simulink model "RobotArmVersion4Assem"  (R2025b)
(part 2 of 11)

  Cylindrical22/LConn1 -- Robot_Arm_2_Version_4_1_RIGID/RConn4
  Cylindrical22/RConn1 -- Motor_Enclosure_Assem_5/LConn1
  Planar18/LConn1 -- Robot_Arm_2_Version_4_1_RIGID/RConn2
  Planar18/RConn1 -- SS_joint_shaft_3_Quarter_Diameter_1_RIGID/LConn2
  x18_Tooth_Timing_Belt_Pulley_1326N51_1_RIGID/LConn3 -- x48_Tooth_Timing_Belt_Pulley_1326N63_1_RIGID/LConn2
  Revolute13/LConn1 -- Robot_Arm_1_Curved_Version_4_3_RIGID/RConn17
  Cylindrical3/RConn1 -- x6436K71_Clamping_Two_Piece_Shaft_Collar_3_RIGID/LConn1
  Revolute13/RConn1 -- x18_Tooth_Timing_Belt_Pulley_1326N51_1_RIGID/LConn1
  Tension_belt_mockup_with_tensioner_2_RIGID/LConn2 -- x18_Tooth_Timing_Belt_Pulley_1326N51_1_RIGID/LConn2
  Arm_Hitch_Track_Rod_Prototype_1_RIGID/LConn1 -- Transform1/RConn1
  Cylindrical23/LConn1 -- x98957A184_Grade_B7_Medium_Strength_Steel_Threaded_Rod_1_RIGID/RConn2
  Cylindrical23/RConn1 -- x2796T14_Ultra_Low_Friction_Dry_Running_Thrust_Bearing_1_RIGID/LConn1
  Revolute14/LConn1 -- SS_joint_shaft_3_Quarter_Diameter_1_RIGID/RConn1
  Revolute14/RConn1 -- x6436K72_Clamping_Two_Piece_Shaft_Collar_1_RIGID/LConn2
  Cylindrical24/LConn1 -- SS_joint_shaft_3_Quarter_Diameter_1_RIGID/RConn2
  Cylindrical24/RConn1 -- x6436K72_Clamping_Two_Piece_Shaft_Collar_2_RIGID/LConn1
  Arm_Hitch_Track_Rod_Prototype_1_RIGID/RConn2 -- Planar19/LConn1
  Planar2/LConn1 -- x6436K71_Clamping_Two_Piece_Shaft_Collar_3_RIGID/RConn1
  Arm_Hitch_Track_Rod_Prototype_2_RIGID/LConn2 -- Planar19/RConn1
  Arm_Hitch_Track_Rod_Prototype_1_RIGID/RConn4 -- Planar20/LConn1
  Arm_Hitch_Track_Rod_Prototype_4_RIGID/LConn2 -- Planar20/RConn1
  Arm_Hitch_Track_Rod_Prototype_1_RIGID/RConn3 -- Revolute15/LConn1
  Arm_Base_Mount_Clamp_Motor_Mount_Assem_4_RIGID/LConn2 -- Revolute15/RConn1
  Arm_Hitch_Track_Rod_Prototype_2_RIGID/RConn1 -- Planar21/LConn1
  Arm_Hitch_Track_Rod_Prototype_3_RIGID/LConn2 -- Planar21/RConn1
  Arm_Hitch_Track_Rod_Prototype_2_RIGID/RConn2 -- Cylindrical25/LConn1
  Arm_Base_Mount_Clamp_Motor_Mount_Assem_4_RIGID/LConn1 -- Cylindrical25/RConn1
  Arm_Base_Mount_Clamp_Motor_Mount_Assem_4_RIGID/RConn2 -- Cylindrical26/LConn1
  Planar2/RConn1 -- Robot_Arm_1_Curved_Version_4_3_RIGID/LConn2
  Arm_Hitch_Track_Rod_Prototype_3_RIGID/LConn1 -- Cylindrical26/RConn1
  Arm_Base_Mount_Clamp_Motor_Mount_Assem_4_RIGID/RConn4 -- Cylindrical27/LConn1
  Arm_Hitch_Track_Rod_Prototype_4_RIGID/LConn1 -- Cylindrical27/RConn1
  Arm_Base_Mount_Clamp_Motor_Mount_Assem_4_RIGID/RConn1 -- Cylindrical28/LConn1
  Cylindrical28/RConn1 -- Motor_Enclosure_Assem_6/LConn1
  Planar22/LConn1 -- x6443K42_Single_U_Joint_1_RIGID/RConn1
  Motor_Enclosure_Assem_6/LConn3 -- Planar22/RConn1
  Revolute16/LConn1 -- x98957A184_Grade_B7_Medium_Strength_Steel_Threaded_Rod_1_RIGID/RConn1
  Revolute16/RConn1 -- x6443K42_Single_U_Joint_1_RIGID/LConn1
  Chuck_Mount_Assem_1/RConn1 -- Cylindrical29/LConn1
  Cylindrical4/LConn1 -- SS_joint_shaft_3_RIGID/RConn1
  Cylindrical29/RConn1 -- Robot_Arm_2_Version_4_1_RIGID/LConn1
  Arm_Hitch_Version_4_2_RIGID/RConn19 -- Cylindrical30/LConn1
  Cylindrical30/RConn1 -- Motor_Enclosure_Assem_4/LConn3
  Revolute17/LConn1 -- x48_Tooth_Timing_Belt_Pulley_1326N63_1_RIGID/RConn1
  Revolute17/RConn1 -- Tension_belt_mockup_with_tensioner_2_RIGID/LConn1
  Arm_Hitch_Version_4_2_RIGID/RConn22 -- Planar23/LConn1
  Planar23/RConn1 -- x6436K71_Clamping_Two_Piece_Shaft_Collar_8_RIGID/LConn2
  Arm_Hitch_Version_4_2_RIGID/RConn23 -- Planar24/LConn1
  Planar24/RConn1 -- SS_joint_shaft_1_RIGID/LConn2
  Arm_Hitch_Version_4_2_RIGID/RConn7 -- Planar25/LConn1
  Cylindrical4/RConn1 -- x6436K71_Clamping_Two_Piece_Shaft_Collar_4_RIGID/LConn2
  Planar25/RConn1 -- SS_joint_shaft_2_RIGID/LConn1
  Arm_Hitch_Version_4_2_RIGID/RConn5 -- Planar26/LConn1
  Planar26/RConn1 -- SS_joint_shaft_3_RIGID/LConn1
  Arm_Hitch_Version_4_2_RIGID/RConn6 -- Planar27/LConn1
  Planar27/RConn1 -- SS_joint_shaft_4_RIGID/LConn2
  Arm_Hitch_Version_4_2_RIGID/RConn4 -- Revolute18/LConn1
  Revolute18/RConn1 -- SS_joint_shaft_5_RIGID/LConn1
  Arm_Hitch_Version_4_2_RIGID/RConn3 -- Planar28/LConn1
  Planar28/RConn1 -- x6436K71_Clamping_Two_Piece_Shaft_Collar_11_RIGID/LConn2
  Arm_Hitch_Version_4_2_RIGID/RConn1 -- Revolute19/LConn1
  Planar3/LConn1 -- x1258N17_11_8_OD_PEEK_Plastic_Ball_Bearing_1_RIGID/RConn1
  Revolute19/RConn1 -- Robot_Arm_1_Curved_Version_4_3_RIGID/LConn1
  Arm_Hitch_Version_4_2_RIGID/RConn2 -- Planar29/LConn1
  Motor_Enclosure_Assem_4/LConn1 -- Planar29/RConn1
  Arm_Hitch_Version_4_2_RIGID/RConn21 -- Revolute20/LConn1
  Revolute20/RConn1 -- x1258N23_15_8_OD_PEEK_Plastic_Ball_Bearing_4_RIGID/LConn1
  Revolute21/LConn1 -- x9533T3_Self_Aligning_Linear_Sleeve_Bearing_1_RIGID/RConn1
  Arm_Hitch_Version_4_2_RIGID/LConn2 -- Revolute21/RConn1
  Arm_Hitch_Version_4_2_RIGID/RConn20 -- Revolute22/LConn1
  Revolute22/RConn1 -- x9533T3_Self_Aligning_Linear_Sleeve_Bearing_2_RIGID/LConn1
  Arm_Hitch_Version_4_2_RIGID/RConn18 -- Revolute23/LConn1
  Planar3/RConn1 -- x6436K71_Clamping_Two_Piece_Shaft_Collar_4_RIGID/LConn1
  Revolute23/RConn1 -- x9533T3_Self_Aligning_Linear_Sleeve_Bearing_3_RIGID/LConn1
  Arm_Hitch_Version_4_2_RIGID/RConn17 -- Revolute24/LConn1
  Revolute24/RConn1 -- x9533T3_Self_Aligning_Linear_Sleeve_Bearing_4_RIGID/LConn1
  Arm_Hitch_Version_4_2_RIGID/RConn16 -- Revolute25/LConn1
  Revolute25/RConn1 -- x9533T3_Self_Aligning_Linear_Sleeve_Bearing_5_RIGID/LConn1
  Arm_Hitch_Version_4_2_RIGID/RConn14 -- Revolute26/LConn1
  Revolute26/RConn1 -- x9533T3_Self_Aligning_Linear_Sleeve_Bearing_6_RIGID/LConn1
  Arm_Hitch_Version_4_2_RIGID/RConn12 -- Revolute27/LConn1
  Revolute27/RConn1 -- x9533T3_Self_Aligning_Linear_Sleeve_Bearing_7_RIGID/LConn1
  Arm_Hitch_Version_4_2_RIGID/RConn11 -- Revolute28/LConn1
  Cylindrical5/LConn1 -- SS_joint_shaft_1_RIGID/RConn2
  Revolute28/RConn1 -- x9533T3_Self_Aligning_Linear_Sleeve_Bearing_8_RIGID/LConn1
  Arm_Hitch_Version_4_2_RIGID/RConn10 -- Revolute29/LConn1
  PEEK_Thread_Insert_1_RIGID/LConn1 -- Revolute29/RConn1
  Arm_Hitch_Version_4_2_RIGID/RConn9 -- Rectangular/LConn1
  Rectangular/RConn1 -- Transform2/RConn1
  Arm_Hitch_Version_4_2_RIGID/RConn8 -- Cylindrical31/LConn1
  Cylindrical31/RConn1 -- Motor_Enclosure_Assem_4/LConn2
  Arm_Hitch_Track_Rod_Prototype_1_RIGID/RConn1 -- Cylindrical32/LConn1
  Arm_Hitch_Version_4_2_RIGID/LConn1 -- Cylindrical32/RConn1
  Arm_Hitch_Version_4_2_RIGID/RConn15 -- Cylindrical33/LConn1
  Cylindrical/RConn1 -- Motor_Enclosure_Assem_5/LConn3
  Cylindrical5/RConn1 -- x6436K71_Clamping_Two_Piece_Shaft_Collar_5_RIGID/LConn1
  Arm_Hitch_Track_Rod_Prototype_2_RIGID/LConn1 -- Cylindrical33/RConn1
  Arm_Hitch_Version_4_2_RIGID/RConn13 -- Revolute30/LConn1
  Arm_Linkage_1_3_RIGID/LConn1 -- Revolute30/RConn1
  Arm_Linkage_1_3_RIGID/RConn2 -- Cylindrical34/LConn1
  Arm_Linkage_2_2_RIGID/LConn2 -- Cylindrical34/RConn1
  Arm_Linkage_1_3_RIGID/RConn1 -- Cylindrical35/LConn1
  Arm_Linkage_2_3_RIGID/LConn2 -- Cylindrical35/RConn1
  Revolute31/LConn1 -- Robot_Arm_1_Curved_Version_4_3_RIGID/RConn12
  Arm_Linkage_2_2_RIGID/LConn1 -- Revolute31/RConn1
  Arm_Linkage_2_2_RIGID/RConn2 -- Revolute32/LConn1
  Planar4/LConn1 -- x6436K71_Clamping_Two_Piece_Shaft_Collar_5_RIGID/RConn1
  Revolute32/RConn1 -- x1258N17_11_8_OD_PEEK_Plastic_Ball_Bearing_3_RIGID/LConn1
  Arm_Linkage_2_2_RIGID/RConn1 -- Revolute33/LConn1
  Revolute33/RConn1 -- x1258N17_11_8_OD_PEEK_Plastic_Ball_Bearing_6_RIGID/LConn1
  Revolute34/LConn1 -- Robot_Arm_1_Curved_Version_4_3_RIGID/RConn11
  Arm_Linkage_2_3_RIGID/LConn1 -- Revolute34/RConn1
  Arm_Linkage_2_3_RIGID/RConn1 -- Revolute35/LConn1
  Revolute35/RConn1 -- x1258N17_11_8_OD_PEEK_Plastic_Ball_Bearing_1_RIGID/LConn1
  Arm_Linkage_2_3_RIGID/RConn2 -- Revolute36/LConn1
  Revolute36/RConn1 -- x1258N17_11_8_OD_PEEK_Plastic_Ball_Bearing_5_RIGID/LConn1
  Planar4/RConn1 -- x1258N17_11_8_OD_PEEK_Plastic_Ball_Bearing_6_RIGID/LConn2
  Cylindrical6/LConn1 -- SS_joint_shaft_1_RIGID/RConn1
  Cylindrical6/RConn1 -- x6436K71_Clamping_Two_Piece_Shaft_Collar_6_RIGID/LConn1
  Planar5/LConn1 -- x6436K71_Clamping_Two_Piece_Shaft_Collar_6_RIGID/RConn1
  Planar5/RConn1 -- x1258N17_11_8_OD_PEEK_Plastic_Ball_Bearing_5_RIGID/LConn2
  Cylindrical7/LConn1 -- SS_joint_shaft_5_RIGID/RConn2
  Cylindrical7/RConn1 -- x6436K71_Clamping_Two_Piece_Shaft_Collar_8_RIGID/LConn1
  Cylindrical8/LConn1 -- SS_joint_shaft_4_RIGID/RConn2
  Cylindrical1/LConn1 -- x6436K71_Clamping_Two_Piece_Shaft_Collar_1_RIGID/RConn1
  Cylindrical8/RConn1 -- x6436K71_Clamping_Two_Piece_Shaft_Collar_9_RIGID/LConn1
  Planar6/LConn1 -- Robot_Arm_1_Curved_Version_4_3_RIGID/RConn16
  Planar6/RConn1 -- x6436K71_Clamping_Two_Piece_Shaft_Collar_9_RIGID/LConn2
  Cylindrical9/LConn1 -- x1258N17_11_8_OD_PEEK_Plastic_Ball_Bearing_6_RIGID/RConn1
  Cylindrical9/RConn1 -- SS_joint_shaft_1_RIGID/LConn1
  Cylindrical10/LConn1 -- x1258N17_11_8_OD_PEEK_Plastic_Ball_Bearing_4_RIGID/RConn1
  Cylindrical10/RConn1 -- SS_joint_shaft_2_RIGID/LConn2
  Cylindrical11/LConn1 -- x1258N17_11_8_OD_PEEK_Plastic_Ball_Bearing_3_RIGID/RConn1
  Cylindrical11/RConn1 -- SS_joint_shaft_3_RIGID/LConn2
  Cylindrical12/LConn1 -- SS_joint_shaft_4_RIGID/RConn1
  Cylindrical1/RConn1 -- SS_joint_shaft_3_RIGID/LConn3
  Cylindrical12/RConn1 -- x6436K71_Clamping_Two_Piece_Shaft_Collar_10_RIGID/LConn1
  Cylindrical13/LConn1 -- Robot_Arm_1_Curved_Version_4_3_RIGID/RConn8
  Cylindrical13/RConn1 -- SS_joint_shaft_4_RIGID/LConn1
  SS_joint_shaft_4_RIGID/LConn3 -- x7749N811_Corrosion_Resistant_Extension_Spring_with_Loop_Ends_1_RIGID/LConn2
  Cylindrical14/LConn1 -- SS_joint_shaft_5_RIGID/RConn1
  Cylindrical14/RConn1 -- x6436K71_Clamping_Two_Piece_Shaft_Collar_11_RIGID/LConn1
  SS_joint_shaft_5_RIGID/LConn2 -- x7749N811_Corrosion_Resistant_Extension_Spring_with_Loop_Ends_1_RIGID/LConn1
  Planar7/LConn1 -- Robot_Arm_1_Curved_Version_4_3_RIGID/RConn6
  Planar7/RConn1 -- x6436K71_Clamping_Two_Piece_Shaft_Collar_10_RIGID/LConn2
  Planar8/LConn1 -- Robot_Arm_1_Curved_Version_4_3_RIGID/RConn5
  Planar/LConn1 -- x1258N17_11_8_OD_PEEK_Plastic_Ball_Bearing_3_RIGID/RConn2
  Planar8/RConn1 -- x6436K13_Clamping_Two_Piece_Shaft_Collar_1_RIGID/LConn1
  Cylindrical15/LConn1 -- SS_joint_shaft_3_8th_Diameter_1_RIGID/RConn1
  Cylindrical15/RConn1 -- x6436K13_Clamping_Two_Piece_Shaft_Collar_1_RIGID/LConn2
  Planar9/LConn1 -- x6235K62_Idler_Pulley_1_RIGID/RConn1
  Planar9/RConn1 -- x6436K13_Clamping_Two_Piece_Shaft_Collar_2_RIGID/LConn2
  Revolute/LConn1 -- SS_joint_shaft_3_8th_Diameter_1_RIGID/RConn2
  Revolute/RConn1 -- x6436K13_Clamping_Two_Piece_Shaft_Collar_2_RIGID/LConn1
  Revolute1/LConn1 -- Robot_Arm_1_Curved_Version_4_3_RIGID/RConn18
  Revolute1/RConn1 -- x48_Tooth_Timing_Belt_Pulley_1326N63_1_RIGID/LConn1
  Planar10/LConn1 -- Robot_Arm_2_Version_4_1_RIGID/RConn5
  Planar/RConn1 -- x6436K71_Clamping_Two_Piece_Shaft_Collar_1_RIGID/LConn1
  Planar10/RConn1 -- x48_Tooth_Timing_Belt_Pulley_1326N63_1_RIGID/LConn3
  Planar11/LConn1 -- x48_Tooth_Timing_Belt_Pulley_1326N63_1_RIGID/RConn2
  Planar11/RConn1 -- x6436K72_Clamping_Two_Piece_Shaft_Collar_2_RIGID/LConn2
  Transform/RConn1 -- Work_Area_1_RIGID/LConn1
  Arm_Base_Mount_Clamp_Motor_Mount_Assem_4_RIGID/RConn5 -- Cylindrical16/LConn1
  Cylindrical16/RConn1 -- Motor_Enclosure_Assem_6/LConn4
  Cylindrical17/LConn1 -- Robot_Arm_1_Curved_Version_4_3_RIGID/RConn3
  Cylindrical17/RConn1 -- Motor_Enclosure_Assem_1/LConn2
  Revolute2/LConn1 -- Robot_Arm_1_Curved_Version_4_3_RIGID/RConn2
  Revolute2/RConn1 -- x1258N23_15_8_OD_PEEK_Plastic_Ball_Bearing_1_RIGID/LConn1
  Cylindrical2/LConn1 -- SS_joint_shaft_2_RIGID/RConn2
  Revolute3/LConn1 -- Robot_Arm_1_Curved_Version_4_3_RIGID/RConn7
  Revolute3/RConn1 -- x1258N23_15_8_OD_PEEK_Plastic_Ball_Bearing_2_RIGID/LConn1
  Cylindrical18/LConn1 -- Robot_Arm_1_Curved_Version_4_3_RIGID/RConn1
  Cylindrical18/RConn1 -- Motor_Enclosure_Assem_1/LConn1
  Planar12/LConn1 -- Robot_Arm_1_Curved_Version_4_3_RIGID/RConn4
  Motor_Enclosure_Assem_1/LConn3 -- Planar12/RConn1
  Revolute4/LConn1 -- Robot_Arm_2_Version_4_1_RIGID/RConn1
  Revolute4/RConn1 -- Robot_Arm_1_Curved_Version_4_3_RIGID/LConn3
  Revolute5/LConn1 -- Robot_Arm_1_Curved_Version_4_3_RIGID/RConn15
  Revolute5/RConn1 -- x1258N17_11_8_OD_PEEK_Plastic_Ball_Bearing_2_RIGID/LConn1
  Cylindrical2/RConn1 -- x6436K71_Clamping_Two_Piece_Shaft_Collar_2_RIGID/LConn1
  Revolute6/LConn1 -- Robot_Arm_1_Curved_Version_4_3_RIGID/RConn14
  Revolute6/RConn1 -- x1258N17_11_8_OD_PEEK_Plastic_Ball_Bearing_4_RIGID/LConn1
  Planar13/LConn1 -- Robot_Arm_1_Curved_Version_4_3_RIGID/RConn13
  Planar13/RConn1 -- x7749N811_Corrosion_Resistant_Extension_Spring_with_Loop_Ends_1_RIGID/LConn3
  Revolute7/LConn1 -- Robot_Arm_1_Curved_Version_4_3_RIGID/RConn10
  Revolute7/RConn1 -- x6235K62_Idler_Pulley_1_RIGID/LConn1
  Cylindrical19/LConn1 -- Robot_Arm_1_Curved_Version_4_3_RIGID/RConn9
  Cylindrical19/RConn1 -- SS_joint_shaft_3_8th_Diameter_1_RIGID/LConn1
  Arm_Base_Mount_Clamp_Assem_5_RIGID/RConn1 -- Revolute8/LConn1
  Revolute8/RConn1 -- x2796T14_Ultra_Low_Friction_Dry_Running_Thrust_Bearing_1_RIGID/LConn2
  Planar1/LConn1 -- x1258N17_11_8_OD_PEEK_Plastic_Ball_Bearing_2_RIGID/RConn1
  Arm_Hitch_Track_Rod_Prototype_1_RIGID/RConn5 -- Revolute9/LConn1
  Arm_Base_Mount_Clamp_Assem_5_RIGID/LConn2 -- Revolute9/RConn1
  Arm_Hitch_Track_Rod_Prototype_2_RIGID/RConn3 -- Cylindrical20/LConn1
  Arm_Base_Mount_Clamp_Assem_5_RIGID/LConn1 -- Cylindrical20/RConn1
  Arm_Base_Mount_Clamp_Motor_Mount_Assem_4_RIGID/RConn3 -- Planar14/LConn1
  Motor_Enclosure_Assem_6/LConn2 -- Planar14/RConn1
  Planar15/LConn1 -- Robot_Arm_2_Version_4_1_RIGID/RConn7
  Motor_Enclosure_Assem_5/LConn2 -- Planar15/RConn1
  Planar16/LConn1 -- x1258N23_15_8_OD_PEEK_Plastic_Ball_Bearing_2_RIGID/RConn1
  Planar16/RConn1 -- x6436K72_Clamping_Two_Piece_Shaft_Collar_1_RIGID/LConn1
